simulink model "testingExamples"  (R2019a)
settings: Solver=VariableStepAuto  StartTime=0.0  StopTime=stop_time/2  RelTol=1e-3
values from neighbouring files (symbols this model uses):
  mp = sm_init_avalon_signals(mp)    [sm_callback_init.m]
  Ts = mp.Ts    [sm_compression_init.m]
  X_in = zeros(1, 2^(M_bits+4))    [Compression_Wrapper_V2.m]    (also in Populate_Band_Compression_Lookup_Gain_V2.m = abs(X_in); TestingLibraryScripts.m = X_temp)
libraries: DSP_FPGA_Accelerated_Toolbox x3
settings Model: Creator=Bailey  LastModifiedBy=Bailey

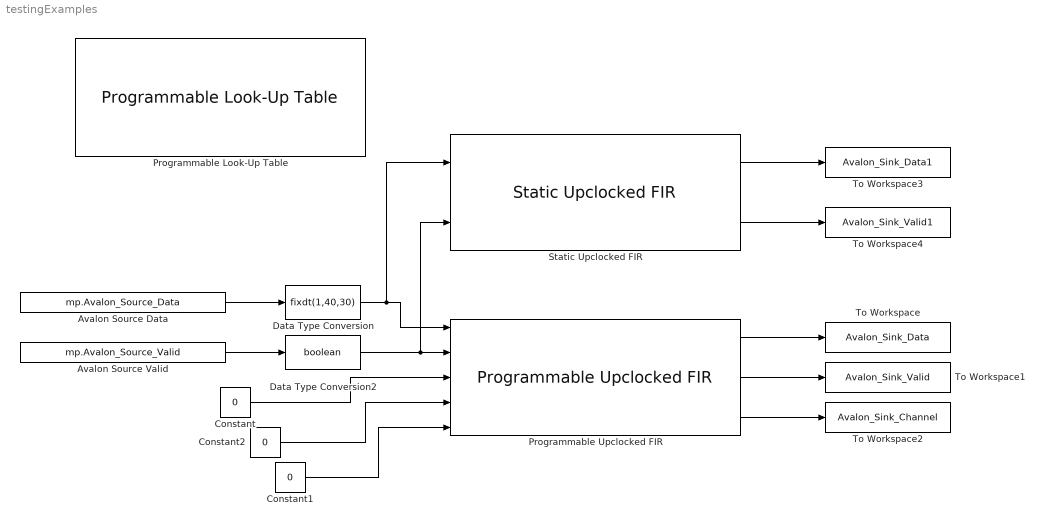
== system testingExamples ==
  "Avalon Source Data " : FromWorkspace  VariableName=mp.Avalon_Source_Data  OutDataTypeStr=double  SampleTime=mp.Ts_system
  Avalon Source Valid : FromWorkspace  VariableName=mp.Avalon_Source_Valid  OutDataTypeStr=double  SampleTime=mp.Ts_system
  Constant : Constant  Value=0  OutDataTypeStr=fixdt(1,34,29)  SampleTime=Ts
  Constant1 : Constant  Value=0  OutDataTypeStr=fixdt(0,2,0)  SampleTime=Ts*3
  Constant2 : Constant  Value=0  OutDataTypeStr=fixdt(0,3,0)  SampleTime=Ts*5
  Data Type Conversion : DataTypeConversion  OutDataTypeStr=fixdt(1,40,30)
  Data Type Conversion2 : DataTypeConversion  OutDataTypeStr=boolean
  Programmable Look-Up Table : DSP_FPGA_Accelerated_Toolbox/Programmable Look-Up Table  TableFn=X_in.^0.5  maxInput=1  floor_in_tab=2^-15  error_cap_tab=0.01  ERR_DIAG=on  N_bits_tab=4  M_bits_tab=5  igotthis=off  Table_Init=0
  Programmable Upclocked FIR : DSP_FPGA_Accelerated_Toolbox/Programmable Upclocked FIR  B_k=[0.5,0.5]  Ts=Ts  Ts_system=Ts_system  Added_Delay=0  W_bits=30  F_bits=20
  Static Upclocked FIR : DSP_FPGA_Accelerated_Toolbox/Static Upclocked FIR  B_k=[0.5,0.5]  Ts=Ts  Ts_system=Ts_system  Added_Delay=0  W_bits=30  F_bits=24
  To Workspace : ToWorkspace  VariableName=Avalon_Sink_Data  SaveFormat=Timeseries  SampleTime=-1
  To Workspace1 : ToWorkspace  VariableName=Avalon_Sink_Valid  SaveFormat=Timeseries  SampleTime=-1
  To Workspace2 : ToWorkspace  VariableName=Avalon_Sink_Channel  SaveFormat=Timeseries  SampleTime=-1
  To Workspace3 : ToWorkspace  VariableName=Avalon_Sink_Data1  SaveFormat=Timeseries  SampleTime=-1
  To Workspace4 : ToWorkspace  VariableName=Avalon_Sink_Valid1  SaveFormat=Timeseries  SampleTime=-1
  wires:
  Avalon Source Valid/1 -> Data Type Conversion2/1
  "Avalon Source Data "/1 -> Data Type Conversion/1
  Data Type Conversion/1 -> Static Upclocked FIR/1, Programmable Upclocked FIR/1
  Data Type Conversion2/1 -> Static Upclocked FIR/2, Programmable Upclocked FIR/2
  Constant/1 -> Programmable Upclocked FIR/3
  Programmable Upclocked FIR/1 -> To Workspace/1
  Programmable Upclocked FIR/2 -> To Workspace1/1
  Programmable Upclocked FIR/3 -> To Workspace2/1
  Constant1/1 -> Programmable Upclocked FIR/5
  Constant2/1 -> Programmable Upclocked FIR/4
  Static Upclocked FIR/2 -> To Workspace4/1
  Static Upclocked FIR/1 -> To Workspace3/1
